simulink model "verify_Room_Node_mdl"  (R2016b)
settings: Solver=ode15s  StartTime=0  StopTime=24*3600  MaxStep=60  RelTol=1e-3  EnableMultiTasking=on
libraries: carnot x4, simulink x1
settings Model: Creator=drhf  LastModifiedBy=drhf
settings DataIOCC: SaveFormat=Array  SignalLoggingSaveFormat=ModelDataLogs
settings OptimizationCC: ExpressionDepthLimit=2147483647  LifeSpan=inf
settings DebuggingCC: UnderspecifiedInitializationDetection=Classic  MergeDetectMultiDrivingBlocksExec=none  SolverPrmCheckMsg=warning  FcnCallInpInsideContextMsg=warning  StateNameClashWarn=warning  SFUnexpectedBacktrackingDiag=warning  SFNoUnconditionalDefaultTransitionDiag=warning  SFExecutionAtInitializationDiag=none
settings HardwareCC: ProdBitPerPointer=32  ProdBitPerSizeT=32  ProdBitPerPtrDiffT=32  ProdLargestAtomicFloat=None  ProdIntDivRoundTo=Undefined  ProdEndianess=Unspecified  ProdWordSize=32  ProdHWDeviceType=32-bit Generic
settings ModelReferenceCC: PropagateSignalLabelsOutOfModel=off
settings GRTTargetCC: TargetLangStandard=C89/C90 (ANSI)  GeneratePreprocessorConditionals=Disable all  CombineOutputUpdateFcns=off  GRTInterface=on
settings ConfigComp: CovMetricSettings=dw  CovHtmlReporting=on  CovSaveCumulativeToWorkspaceVar=on  CovSaveSingleToWorkspaceVar=on  CovExternalEMLEnable=off

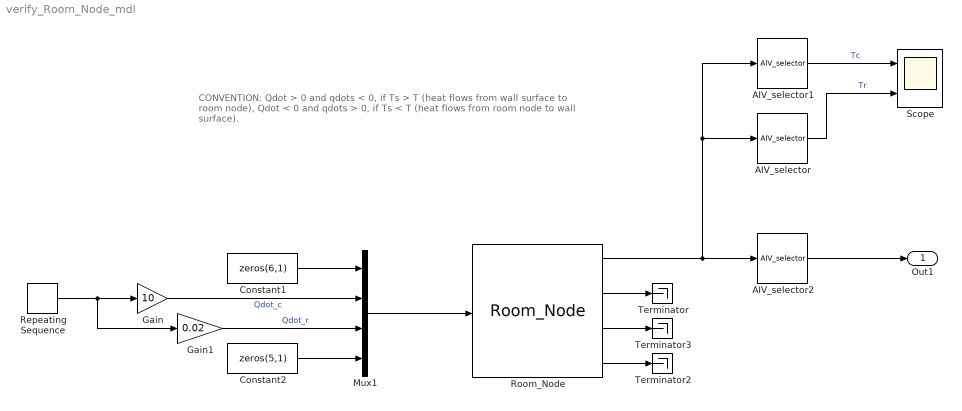
== system verify_Room_Node_mdl ==
  note: CONVENTION:
      | Qdot > 0 and qdots < 0, if Ts > T (heat flows from wall surface to room node),
      | Qdot < 0 and qdots > 0, if Ts < T (heat flows from room node to wall surface).
  AIV_selector : carnot/Outputs/AIV_selector  e1=off  e2=off  e3=on  e4=off  e5=off  e6=off  e7=off  e8=off  e9=off
  AIV_selector1 : carnot/Outputs/AIV_selector  e1=off  e2=on  e3=off  e4=off  e5=off  e6=off  e7=off  e8=off  e9=off
  AIV_selector2 : carnot/Outputs/AIV_selector  e1=off  e2=on  e3=on  e4=off  e5=off  e6=off  e7=off  e8=off  e9=off
  Constant1 : Constant  Value=zeros(6,1)
  Constant2 : Constant  Value=zeros(5,1)
  Gain : Gain  Gain=10
  Gain1 : Gain  Gain=0.02
  Mux1 : Mux  Inputs=[6 1 1 5]
  Repeating Sequence : simulink/Sources/Repeating Sequence  rep_seq_t=[0 12 12.001 24.1]*3600  rep_seq_y=[-1 -1 1 1]
  Room_Node : carnot/Load/Houses/room_nodes/Room_Node  zoneairvolume=5*5*2.5  zoneheight=2.5  zonestartTEMP=22  zonestartWATER=50  timeconst=100  heatperfect=natural  lookuptime=[0 24]*3600  lookupvalue=[20 20]  AirPressure=101300
  Scope : Scope  NumInputPorts=2
  Terminator : Terminator
  Terminator2 : Terminator
  Terminator3 : Terminator
  Out1 : Outport
  wires:
  AIV_selector/1 -> Scope/2  "Tr"
  Room_Node/2 -> Terminator/1
  Room_Node/4 -> Terminator2/1
  Room_Node/3 -> Terminator3/1
  Room_Node/1 -> AIV_selector2/1, AIV_selector1/1, AIV_selector/1
  Mux1/1 -> Room_Node/1
  Constant2/1 -> Mux1/4
  Constant1/1 -> Mux1/1
  Gain/1 -> Mux1/2  "Qdot_c"
  Gain1/1 -> Mux1/3  "Qdot_r"
  Repeating Sequence/1 -> Gain1/1, Gain/1
  AIV_selector1/1 -> Scope/1  "Tc"
  AIV_selector2/1 -> Out1/1
